simulink model "Simulatoin_Model"  (R2020b)
settings: Solver=ode45  StartTime=0.0  StopTime=100.0  MaxStep=0.01  RelTol=1e-6
settings Model: Creator=edward  LastModifiedBy=edward

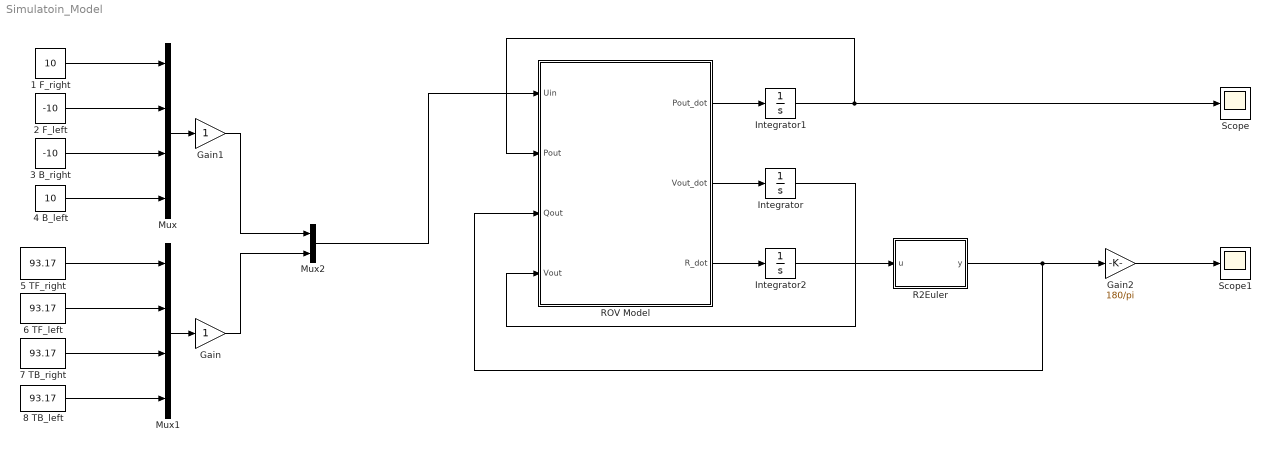
== system Simulatoin_Model ==
  1 F_right : Constant  Value=10
  2 F_left : Constant  Value=-10
  3 B_right : Constant  Value=-10
  4 B_left : Constant  Value=10
  5 TF_right : Constant  Value=93.17
  6 TF_left : Constant  Value=93.17
  7 TB_right : Constant  Value=93.17
  8 TB_left : Constant  Value=93.17
  Gain : Gain
  Gain1 : Gain
  Gain2 : Gain  Gain=180/pi
  Integrator : Integrator  InitialCondition=zeros(6,1)
  Integrator1 : Integrator  InitialCondition=zeros(3,1)
  Integrator2 : Integrator  InitialCondition=eye(3)
  Mux : Mux
  Mux1 : Mux
  Mux2 : Mux  Inputs=2
  R2Euler : MATLAB Function  TreatAsAtomicUnit=on
  ROV Model : MATLAB Function  TreatAsAtomicUnit=on
  Scope : Scope
  Scope1 : Scope
  wires:
  ROV Model/2(Vout_dot) -> Integrator/1
  1 F_right/1 -> Mux/1
  4 B_left/1 -> Mux/4
  3 B_right/1 -> Mux/3
  2 F_left/1 -> Mux/2
  6 TF_left/1 -> Mux1/2
  7 TB_right/1 -> Mux1/3
  8 TB_left/1 -> Mux1/4
  Mux/1 -> Gain1/1
  Mux1/1 -> Gain/1
  Mux2/1 -> ROV Model/1(Uin)
  Gain/1 -> Mux2/2
  5 TF_right/1 -> Mux1/1
  Integrator/1 -> ROV Model/4(Vout)
  ROV Model/1(Pout_dot) -> Integrator1/1
  Gain1/1 -> Mux2/1
  Integrator1/1 -> Scope/1, ROV Model/2(Pout)
  ROV Model/3(R_dot) -> Integrator2/1
  Integrator2/1 -> R2Euler/1(u)
  R2Euler/1(y) -> Gain2/1, ROV Model/3(Qout)
  Gain2/1 -> Scope1/1

== matlab function Simulatoin_Model/ROV Model ==
  data: Uin input size=8; Pout_dot output size=3; Pout input size=3; Qout input size=3; Vout_dot output size=6; Vout input size=6; R_dot output size=[3 3]
function [Pout_dot,Vout_dot,R_dot] = fcn(Uin,Pout,Qout,Vout)

pos = Pout(1:3);

roll = Qout(1);
pitch = Qout(2);
yaw = Qout(3);

v_surge = Vout(1);
v_sway = Vout(2);
v_heave = Vout(3);
w_roll = Vout(4);
w_pitch = Vout(5);
w_yaw = Vout(6);

v1 = [v_surge v_sway v_heave]';
v2 = [w_roll w_pitch w_yaw]';


L1 = .20;
L2 = .15;
L3 = .15;
L4 = .15;
L5 = .05;
L6 = (L2^2 + L4^2)^0.5;
L7 = (L3^2 + L4^2)^0.5;
L8 = (L1^2 + L5^2)^0.5;
L9 = (L2^2 + L5^2)^0.5;
L10 = (L3^2 + L5^2)^0.5;
theta1 = atan(L4/L2);
theta2 = atan(L4/L3);
theta3 = atan(L5/L1);
theta4 = atan(L5/L2);
theta5 = atan(L5/L3);
L = [-(1/2)^(-1/2) -(1/2)^(-1/2) (1/2)^(-1/2)  (1/2)^(-1/2) 0 0 0 0;
      (1/2)^(-1/2) -(1/2)^(-1/2) (1/2)^(-1/2) -(1/2)^(-1/2) 0 0 0 0;
     0 0 0 0 1 1 1 1;
     0 0 0 0  L8*cos(theta3) -L8*cos(theta3)  L8*cos(theta3) -L8*cos(theta3);
     0 0 0 0 -L9*cos(theta4) -L9*cos(theta4)  L10*cos(theta5)  L10*cos(theta5);
     L6*cos(pi/4-theta1) -L6*cos(pi/4-theta1) -L7*cos(pi/4-theta2) L7*cos(pi/4-theta2) 0 0 0 0];
tor = L*Uin;

X_u = 10;
Y_v = 10;
Z_w = 10;
K_p = 10;
M_q = 10;
N_r = 10;
r_g = [0 0 0]';
I_g = diag([0.13, 0.16, 0.2]);
m = 10;

MRB = [m*eye(3) -m*Skew(r_g);
       m*Skew(r_g) I_g];
   
MA = diag([X_u, Y_v, Z_w, K_p, M_q, N_r]);
  
M = MRB + MA;

CRB = [zeros(3,3), -m*Skew(v1)-m*Skew(Skew(v2)*r_g);
       -m*Skew(v1)-m*Skew(Skew(v2)*r_g) m*Skew(Skew(v1)*r_g)-Skew(I_g*v2)];
   
a1 = X_u*v_surge;
a2 = Y_v*v_sway;
a3 = Z_w*v_heave;
b1 = K_p*w_roll;
b2 = M_q*w_pitch;
b3 = N_r*w_yaw;

aux_a = [a1; a2; a3];
aux_b = [b1; b2; b3];

CA = [  zeros(3,3), Skew(aux_a);
        Skew(aux_a), Skew(aux_b)];
    
C = CRB + CA;

Xu = 10;
Yv = 10;
Zw = 10;
Kp = 10;
Mq = 10;
Nr = 10;
Xuu = 10;
Yvv = 10;
Zww = 10;
Kpp = 10;
Mqq = 10;
Nrr = 10;  
Dl = diag([Xu, Yv, Zw, Kp, Mq, Nr]);
Dq = diag([Xuu*abs(v_surge), Yvv*abs(v_sway), Zww*abs(v_heave), Kpp*abs(w_roll), Mqq*abs(w_pitch), Nrr*abs(w_yaw)]);
D = Dl + Dq;

W = 9.81*m;
B = 1000*9.81*0.0480;
g = [(W-B)*sin(pitch);
     -(W-B)*cos(pitch)*sin(roll);
     -(W-B)*cos(pitch)*cos(roll);
     0;
     0;
     0];

% R = Rzyx(roll, pitch, yaw);
% T = [1 sin(roll)*tan(pitch) cos(roll)*tan(pitch);
%      0 cos(roll)            -sin(roll);
%      0 sin(roll)/cos(pitch) cos(roll)/cos(pitch)];
% J = [R zeros(3);
%     zeros(3) T];
% 
% Pout_dot = J*Vout;

% w_pitch = euler2q(roll, pitch, yaw);
% [J, J11, J22] = quatern(w_pitch);
% 
% p_dot = J11*v1;
% q_dot = J22*v2;
% 
% euler_angles = quat2eul(q_dot'/norm(q_dot));
% Pout_dot = [p_dot(1) p_dot(2) p_dot(3) euler_angles(1) euler_angles(2) euler_angles(3)]';

R = eul2rotm([roll, pitch, yaw], 'XYZ');
Pout_dot = R*v1;

R_dot = R*Skew(v2);

Vout_dot = M\(tor - C*Vout - D*Vout - g);

== matlab function Simulatoin_Model/R2Euler ==
  data: u input; y output
function y = fcn(u)
y = rotm2eul(u, 'XYZ')';
